simulink model "PubIfDecisionLM_MDL"  (R2020b)
settings: configuration reference "DspaceConfig" (kept outside this file)
PostLoadFcn:
  | if any(exist('dsrtsu_mdlpostloadfcn', 'file') ~= 0), dsrtsu_mdlpostloadfcn('Execute', bdroot); end
InitFcn:
  | , if any(exist('dsmpb_private', 'file') ~= 0), dsmpb_private('dsmpb_mdlclblib', 'Init', bdroot); end,
undefined symbols (not defined in the file or in its folder): OFM_OBJ_FUSIONTYPE_E, OFM_OBJ_MOVINGSTATE_E, OFM_OBJ_ORIENTATION_E, OFM_OBJ_TYPE_E, P_LM_Cyc, P_LM_EMLHistKapRcdBufSize, P_LM_EMLHistTrajBaseDis, P_LM_EMLHistTrajPNum, P_LM_EMLKapCorrMaxThre, P_LM_EMLMinKapThre, P_LM_EMLPathDisDiffThre, P_LM_EMLQuaFiltPar, P_LM_EMLTurnActKapThre, P_LM_EMLValidQuaThre, P_LM_FntPath1Disgap, P_LM_FntPath1MinDis, P_LM_FntPath1Timegap, P_LM_FntPath2Disgap, P_LM_FntPath2MinDis, P_LM_FntPath2Timegap, P_LM_FntPath3Disgap, P_LM_FntPath3MinDis, P_LM_FntPath3Timegap, P_LM_FusBLParFiltP, P_LM_FusEVDifC2Thre, P_LM_FusEVOPath1AllVSLDisThre, P_LM_FusEVOPath1AllVSLLostNumThre, P_LM_FusEVOPath1AllVSLQuaThre, P_LM_FusEVOPath1OTLFacNLC, P_LM_FusOTLQuaThre, P_LM_FusOTLSW, P_LM_FusParC0Index, P_LM_FusParC1Index, P_LM_FusParC2Index, P_LM_FusParC3Index, P_LM_FusVSLQuaThre, P_LM_FusVSLSW, P_LM_FusVSLValidSteerWheerAngThre, P_LM_FusVSLValidVxvThre, P_LM_LaneWidth, P_LM_OTLBufTPInfoEvaFactor, P_LM_OTLObjNum, P_LM_OTLObjSelectAgeThre, P_LM_OTLObjSelectDxAssessVx, P_LM_OTLObjSelectDxThre, P_LM_OTLObjSelectVxThre, P_LM_OTLObjSelectVyAssessDx, P_LM_OTLObjSelectVyThre, P_LM_OTLTrajPntBaseDis, P_LM_OTLTrajStdThre, P_LM_VSLAvailLineNum, P_LM_VSLBLSDiffThre, P_LM_VSLBLSDisRatio, P_LM_VSLFusBLParFiltP_C1, P_LM_VSLFusBLParFiltP_C2, P_LM_VSLFusBLParFiltP_C3, P_LM_VSLFusBLParFiltP_Quality, P_LM_VSLHistTrajBaseDis, P_LM_VSLHistTrajPNum, P_LM_VSLLCC0diff ... (+18)
libraries: simulink x145, LM_LIB x43
(part 17 of 24)

== system PubIfDecisionLM_MDL/Subsystem2/LM_Fusion1/LM_FusRatioCalc/LM_Fusion_EVO/LM_FusEVORatioCalc/LM_Fusion_FntPathK/LM_FusEVOFntPath1/LM_FUS_EVOFEMLKAdju ==
  LM_EMLFntPath1Quality : Inport
  DIR_LC2LeValid : Inport  Port=2
  DIR_LC2RigValid : Inport  Port=3
  vxvRefMs : Inport  Port=4
  LM_FusEVOFntPath1EMLKBefAdju : Inport  Port=5
  LM_FusEVOFntPath1VSLKBefAdju : Inport  Port=6
  LM_FusEVOFntPath1OTLKBefAdju : Inport  Port=7
  Add : Sum
  Compare To Zero : simulink/Logic and Bit Operations/Compare To Zero  relop===  OutDataTypeStr=boolean
  Constant : Constant  Value=0.000001  OutDataTypeStr=single
  Constant1 : Constant  OutDataTypeStr=single
  Constant2 : Constant  Value=10  OutDataTypeStr=single
  Constant3 : Constant  Value=6  OutDataTypeStr=single
  Constant4 : Constant  Value=0.6  OutDataTypeStr=single
  Constant5 : Constant  Value=0.45  OutDataTypeStr=single
  Constant7 : Constant  Value=0.6
  Divide : Product  Inputs=*/
  Divide1 : Product  Inputs=*/
  Logical Operator : Logic  AllPortsSameDT=off  OutDataTypeStr=boolean
  Logical Operator1 : Logic  AllPortsSameDT=off  OutDataTypeStr=boolean
  Logical Operator2 : Logic  Operator=OR  AllPortsSameDT=off  OutDataTypeStr=boolean
  Logical Operator3 : Logic  Operator=NOT  AllPortsSameDT=off  OutDataTypeStr=boolean
  Logical Operator4 : Logic  AllPortsSameDT=off  OutDataTypeStr=boolean
  Max : MinMax  Function=max  Inputs=2
  Max1 : MinMax  Function=max  Inputs=2
  Product : Product
  Product1 : Product
  Relational Operator1 : RelationalOperator  OutDataTypeStr=boolean  RndMeth=Simplest
  Relational Operator2 : RelationalOperator  OutDataTypeStr=boolean  RndMeth=Simplest
  Relational Operator3 : RelationalOperator  OutDataTypeStr=boolean  RndMeth=Simplest
  Subtract : Sum  Inputs=+-
  Switch{,1..4} (5 alike) : Switch  Criteria=u2 ~= 0
  LM_FusEVOFntPath1EMLK : Outport
  LM_FusEVOFntPath1VSLK : Outport  Port=2
  LM_FusEVOFntPath1OTLK : Outport  Port=3
  wires:
  Relational Operator2/1 -> Logical Operator1/2
  Relational Operator1/1 -> Logical Operator/2
  Logical Operator4/1 -> Logical Operator/1, Logical Operator1/1
  Constant7/1 -> Relational Operator3/2
  Max1/1 -> Switch2/1
  Constant5/1 -> Max1/2
  Switch2/1 -> Switch1/3
  Max/1 -> Switch1/1
  LM_FusEVOFntPath1EMLKBefAdju/1 -> Switch2/3, Max1/1, Max/1
  Constant4/1 -> Max/2
  Logical Operator1/1 -> Switch4/2, Switch3/2, Switch2/2
  Constant3/1 -> Relational Operator2/2
  Logical Operator/1 -> Switch1/2
  Constant2/1 -> Relational Operator1/2
  vxvRefMs/1 -> Relational Operator1/1, Relational Operator2/1
  LM_EMLFntPath1Quality/1 -> Relational Operator3/1
  Switch1/1 -> LM_FusEVOFntPath1EMLK/1, Subtract/2  "LM_FusEOFntPath1EMLK"
  DIR_LC2LeValid/1 -> Logical Operator2/1
  DIR_LC2RigValid/1 -> Logical Operator2/2
  Logical Operator2/1 -> Logical Operator3/1
  Logical Operator3/1 -> Logical Operator4/1
  Relational Operator3/1 -> Logical Operator4/2
  LM_FusEVOFntPath1VSLKBefAdju/1 -> Add/1, Switch3/3, Divide/1
  LM_FusEVOFntPath1OTLKBefAdju/1 -> Divide1/1, Switch4/3, Add/2
  Add/1 -> Switch/3, Compare To Zero/1
  Compare To Zero/1 -> Switch/2
  Constant/1 -> Switch/1
  Switch/1 -> Divide/2, Divide1/2
  Constant1/1 -> Subtract/1
  Subtract/1 -> Product1/1, Product/1
  Divide/1 -> Product/2
  Product/1 -> Switch3/1
  Product1/1 -> Switch4/1
  Divide1/1 -> Product1/2
  Switch3/1 -> LM_FusEVOFntPath1VSLK/1  "LM_FusEVOFntPath1VSLK"
  Switch4/1 -> LM_FusEVOFntPath1OTLK/1  "LM_FusEVOFntPath1OTLK"

== system PubIfDecisionLM_MDL/Subsystem2/LM_Fusion1/LM_FusRatioCalc/LM_Fusion_EVO/LM_FusEVORatioCalc/LM_Fusion_FntPathK/LM_FusEVOFntPath1/LM_FusEVOFntPath1AllEML ==
  Action Port : ActionPort  ActionPortLabel=elseif(u1 ==2)
  Constant : Constant  OutDataTypeStr=single
  Constant1 : Constant  Value=0  OutDataTypeStr=single
  Constant2 : Constant  Value=0  OutDataTypeStr=single
  LM_FusEVOFntPath1EMLK : Outport
  LM_FusEVOFntPath1VSLK : Outport  Port=2
  LM_FusEVOFntPath1OTLK : Outport  Port=3
  wires:
  Constant/1 -> LM_FusEVOFntPath1EMLK/1
  Constant2/1 -> LM_FusEVOFntPath1OTLK/1
  Constant1/1 -> LM_FusEVOFntPath1VSLK/1

== system PubIfDecisionLM_MDL/Subsystem2/LM_Fusion1/LM_FusRatioCalc/LM_Fusion_EVO/LM_FusEVORatioCalc/LM_Fusion_FntPathK/LM_FusEVOFntPath1/LM_FusEVOFntPath1AllVSL ==
  Action Port : ActionPort  ActionPortLabel=if(u1 == 1)
  Constant : Constant  Value=0  OutDataTypeStr=single
  Constant1 : Constant  OutDataTypeStr=single
  Constant2 : Constant  Value=0  OutDataTypeStr=single
  LM_FusEVOFntPath1EMLK : Outport
  LM_FusEVOFntPath1VSLK : Outport  Port=2
  LM_FusEVOFntPath1OTLK : Outport  Port=3
  wires:
  Constant/1 -> LM_FusEVOFntPath1EMLK/1
  Constant1/1 -> LM_FusEVOFntPath1VSLK/1
  Constant2/1 -> LM_FusEVOFntPath1OTLK/1

== system PubIfDecisionLM_MDL/Subsystem2/LM_Fusion1/LM_FusRatioCalc/LM_Fusion_EVO/LM_FusEVORatioCalc/LM_Fusion_FntPathK/LM_FusEVOFntPath1/LM_FusEVO_AllVSLJudge ==
  note: 0 Fus
      | 1 All VSL
      | 2 All EML
  note: 完全用车道线场景：当车道线很好的时候可以完全用车道线，否则为了增加道路模型鲁棒性对三个道路模型加权平均
      | 1. 丢失车道数<=1
      | 2. 车道线质量大于0.65
      | 3. 第一段道路模型距离-VSL基础距离<=8m
  LM_VSLBaseDis : Inport
  LM_ComLineLostNum : Inport  Port=2
  LM_FntPath1Dis : Inport  Port=3
  DIR_TurnLeftValid : Inport  Port=4
  DIR_TurnRightValid : Inport  Port=5
  LM_VSLFntPath1Quality : Inport  Port=6
  Constant : Constant  Value=P_LM_FusEVOPath1AllVSLLostNumThre  OutDataTypeStr=uint8
  Constant1 : Constant  Value=P_LM_FusEVOPath1AllVSLQuaThre  OutDataTypeStr=single
  Constant2 : Constant  Value=P_LM_FusEVOPath1AllVSLDisThre  OutDataTypeStr=single
  Constant3 : Constant  OutDataTypeStr=uint8
  Constant4 : Constant  Value=0  OutDataTypeStr=uint8
  Constant5 : Constant  Value=2  OutDataTypeStr=uint8
  Logical Operator : Logic  Inputs=3  AllPortsSameDT=off  OutDataTypeStr=boolean
  Logical Operator1 : Logic  Operator=OR  AllPortsSameDT=off  OutDataTypeStr=boolean
  Relational Operator : RelationalOperator  Operator=<=  OutDataTypeStr=boolean  RndMeth=Simplest
  Relational Operator1 : RelationalOperator  OutDataTypeStr=boolean  RndMeth=Simplest
  Relational Operator2 : RelationalOperator  Operator=<=  OutDataTypeStr=boolean  RndMeth=Simplest
  Subtract : Sum  Inputs=+-
  Switch : Switch  Criteria=u2 ~= 0
  Switch1 : Switch  Criteria=u2 ~= 0
  LM_FusEVOFusType : Outport
  wires:
  LM_ComLineLostNum/1 -> Relational Operator/1
  Constant/1 -> Relational Operator/2
  LM_VSLFntPath1Quality/1 -> Relational Operator1/1
  Constant1/1 -> Relational Operator1/2
  LM_VSLBaseDis/1 -> Subtract/2
  LM_FntPath1Dis/1 -> Subtract/1
  Subtract/1 -> Relational Operator2/1
  Constant2/1 -> Relational Operator2/2
  Relational Operator1/1 -> Logical Operator/1
  Relational Operator/1 -> Logical Operator/2
  Relational Operator2/1 -> Logical Operator/3
  Logical Operator/1 -> Switch1/2  "LM_FusEVOAllVSLflg"
  DIR_TurnLeftValid/1 -> Logical Operator1/1
  DIR_TurnRightValid/1 -> Logical Operator1/2
  Logical Operator1/1 -> Switch/2  "LM_FusEVOAllEMLflg"
  Switch/1 -> LM_FusEVOFusType/1  "LM_FusEVOFusType"
  Constant3/1 -> Switch1/1
  Constant4/1 -> Switch1/3
  Switch1/1 -> Switch/3
  Constant5/1 -> Switch/1

== system PubIfDecisionLM_MDL/Subsystem2/LM_Fusion1/LM_FusRatioCalc/LM_Fusion_EVO/LM_FusEVORatioCalc/LM_Fusion_FntPathK/LM_FusEVOFntPath2/If Action Subsystem ==
  Action Port : ActionPort  ActionPortLabel=if(u1 == 1)
  Constant : Constant  Value=0  OutDataTypeStr=single
  Constant1 : Constant  OutDataTypeStr=single
  Constant2 : Constant  Value=0  OutDataTypeStr=single
  LM_FusEVOFntPath2EMLK : Outport
  LM_FusEVOFntPath2VSLK : Outport  Port=2
  LM_FusEVOFntPath2OTLK : Outport  Port=3
  wires:
  Constant2/1 -> LM_FusEVOFntPath2OTLK/1
  Constant1/1 -> LM_FusEVOFntPath2VSLK/1
  Constant/1 -> LM_FusEVOFntPath2EMLK/1

== system PubIfDecisionLM_MDL/Subsystem2/LM_Fusion1/LM_FusRatioCalc/LM_Fusion_EVO/LM_FusEVORatioCalc/LM_Fusion_FntPathK/LM_FusEVOFntPath2/If Action Subsystem1 ==
  LM_EMLFntPath2Quality : Inport
  LM_VSLFntPath2Quality : Inport  Port=2
  LM_OTLFntPath2Qulity : Inport  Port=3
  vxvRefMs : Inport  Port=4
  DIR_LC2LeValid : Inport  Port=5
  DIR_LC2RigValid : Inport  Port=6
  Action Port : ActionPort  ActionPortLabel=else
  LM_FusEVO_EMLFactor : Subsystem
  LM_FusEVO_OTLFactor : Subsystem
  LM_FusEVO_VSLFactor : Subsystem
  Subsystem : Subsystem
  LM_FusEVOFntPath2EMLK : Outport
  LM_FusEVOFntPath2VSLK : Outport  Port=2
  LM_FusEVOFntPath2OTLK : Outport  Port=3
  wires:
  Subsystem/1(LM_FusEVOFntPath2EMLK) -> LM_FusEVOFntPath2EMLK/1  "LM_FusEVOFntPath2EMLK"
  Subsystem/2(LM_FusEVOFntPath2VSLK) -> LM_FusEVOFntPath2VSLK/1
  Subsystem/3(LM_FusEVOFntPath2OTLK) -> LM_FusEVOFntPath2OTLK/1
  vxvRefMs/1 -> LM_FusEVO_EMLFactor/1(vxvRefMs)
  DIR_LC2LeValid/1 -> LM_FusEVO_OTLFactor/1(DIR_LC2LeValid), LM_FusEVO_EMLFactor/2(DIR_LC2LeValid)
  DIR_LC2RigValid/1 -> LM_FusEVO_OTLFactor/2(DIR_LC2RigValid), LM_FusEVO_EMLFactor/3(DIR_LC2RigValid)
  LM_FusEVO_EMLFactor/1(LM_FusEVOFntPath2EMLFac) -> Subsystem/1(LM_FusEVOFntPath2EMLFac)
  LM_FusEVO_VSLFactor/1(LM_FusEVOFntPath2VSLFac) -> Subsystem/2(LM_FusEVOFntPath2VSLFac)
  LM_FusEVO_OTLFactor/1(LM_FusEVOFntPath2OTLFac) -> Subsystem/3(LM_FusEVOFntPath2OTLFac)
  LM_EMLFntPath2Quality/1 -> Subsystem/4(LM_EMLFntPath2Quality)
  LM_VSLFntPath2Quality/1 -> Subsystem/5(LM_VSLFntPath2Quality)
  LM_OTLFntPath2Qulity/1 -> Subsystem/6(LM_OTLFntPath2Qulity)

== system PubIfDecisionLM_MDL/Subsystem2/LM_Fusion1/LM_FusRatioCalc/LM_Fusion_EVO/LM_FusEVORatioCalc/LM_Fusion_FntPathK/LM_FusEVOFntPath2/If Action Subsystem2 ==
  Action Port : ActionPort  ActionPortLabel=elseif(u1 == 2)
  Constant : Constant  OutDataTypeStr=single
  Constant1 : Constant  Value=0  OutDataTypeStr=single
  Constant2 : Constant  Value=0  OutDataTypeStr=single
  LM_FusEVOFntPath2EMLK : Outport
  LM_FusEVOFntPath2VSLK : Outport  Port=2
  LM_FusEVOFntPath2OTLK : Outport  Port=3
  wires:
  Constant/1 -> LM_FusEVOFntPath2EMLK/1
  Constant1/1 -> LM_FusEVOFntPath2VSLK/1
  Constant2/1 -> LM_FusEVOFntPath2OTLK/1

== system PubIfDecisionLM_MDL/Subsystem2/LM_Fusion1/LM_FusRatioCalc/LM_Fusion_EVO/LM_FusEVORatioCalc/LM_Fusion_FntPathK/LM_FusEVOFntPath2/LM_FusEVO_AllVSLJudge ==
  note: 完全用车道线场景：当车道线很好的时候可以完全用车道线，否则为了增加道路模型鲁棒性对三个道路模型加权平均
      | 1. 丢失车道数<=1
      | 2. 车道线质量大于0.65
      | 3. 第一段道路模型距离-VSL基础距离<=8m
  note: 0 Fus
      | 1 All VSL
      | 2 All EML
  LM_ComLineLostNum : Inport
  DIR_TurnLeftValid : Inport  Port=2
  DIR_TurnRightValid : Inport  Port=3
  LM_VSLBaseDis : Inport  Port=4
  LM_FntPath2Dis : Inport  Port=5
  LM_VSLFntPath2Quality : Inport  Port=6
  Constant : Constant  OutDataTypeStr=uint8
  Constant1 : Constant  Value=0.5  OutDataTypeStr=single
  Constant2 : Constant  OutDataTypeStr=uint8
  Constant3 : Constant  Value=0  OutDataTypeStr=uint8
  Constant4 : Constant  Value=8  OutDataTypeStr=single
  Constant5 : Constant  Value=2  OutDataTypeStr=uint8
  Logical Operator : Logic  Inputs=3  AllPortsSameDT=off  OutDataTypeStr=boolean
  Logical Operator1 : Logic  Operator=OR  AllPortsSameDT=off  OutDataTypeStr=boolean
  Relational Operator : RelationalOperator  Operator=<=  OutDataTypeStr=boolean  RndMeth=Simplest
  Relational Operator1 : RelationalOperator  OutDataTypeStr=boolean  RndMeth=Simplest
  Relational Operator2 : RelationalOperator  Operator=<=  OutDataTypeStr=boolean  RndMeth=Simplest
  Subtract : Sum  Inputs=+-
  Switch : Switch  Criteria=u2 ~= 0
  Switch1 : Switch  Criteria=u2 ~= 0
  LM_FusEVOFntPath2FusType : Outport
  wires:
  Logical Operator/1 -> Switch1/2  "LM_FusEVOAllVSLflg"
  Relational Operator/1 -> Logical Operator/2
  Relational Operator1/1 -> Logical Operator/1
  Constant1/1 -> Relational Operator1/2
  LM_VSLFntPath2Quality/1 -> Relational Operator1/1
  Constant/1 -> Relational Operator/2
  LM_ComLineLostNum/1 -> Relational Operator/1
  Constant5/1 -> Switch/1
  Logical Operator1/1 -> Switch/2  "LM_FusEVOAllEMLflg"
  DIR_TurnRightValid/1 -> Logical Operator1/2
  DIR_TurnLeftValid/1 -> Logical Operator1/1
  Switch/1 -> LM_FusEVOFntPath2FusType/1  "LM_FusEVOFntPath2FusType"
  Switch1/1 -> Switch/3
  Constant2/1 -> Switch1/1
  Constant3/1 -> Switch1/3
  Subtract/1 -> Relational Operator2/1
  Constant4/1 -> Relational Operator2/2
  LM_FntPath2Dis/1 -> Subtract/1
  LM_VSLBaseDis/1 -> Subtract/2
  Relational Operator2/1 -> Logical Operator/3

== system PubIfDecisionLM_MDL/Subsystem2/LM_Fusion1/LM_FusRatioCalc/LM_Fusion_EVO/LM_FusEVORatioCalc/LM_Fusion_FntPathK/LM_FusEVOFntPath3/If Action Subsystem ==
  Action Port : ActionPort  ActionPortLabel=if(u1 == 1)
  Constant : Constant  Value=0  OutDataTypeStr=single
  Constant1 : Constant  OutDataTypeStr=single
  Constant2 : Constant  Value=0  OutDataTypeStr=single
  LM_FusEVOFntPath3EMLK : Outport
  LM_FusEVOFntPath3VSLK : Outport  Port=2
  LM_FusEVOFntPath3OTLK : Outport  Port=3
  wires:
  Constant2/1 -> LM_FusEVOFntPath3OTLK/1
  Constant1/1 -> LM_FusEVOFntPath3VSLK/1
  Constant/1 -> LM_FusEVOFntPath3EMLK/1

== system PubIfDecisionLM_MDL/Subsystem2/LM_Fusion1/LM_FusRatioCalc/LM_Fusion_EVO/LM_FusEVORatioCalc/LM_Fusion_FntPathK/LM_FusEVOFntPath3/If Action Subsystem1 ==
  LM_EMLFntPath3Quality : Inport
  LM_VSLFntPath3Quality : Inport  Port=2
  LM_OTLFntPath3Qulity : Inport  Port=3
  vxvRefMs : Inport  Port=4
  DIR_LC2LeValid : Inport  Port=5
  DIR_LC2RigValid : Inport  Port=6
  Action Port : ActionPort  ActionPortLabel=else
  LM_FusEVO_EMLFactor : Subsystem
  LM_FusEVO_OTLFactor : Subsystem
  LM_FusEVO_VSLFactor : Subsystem
  Subsystem : Subsystem
  LM_FusEVOFntPath3EMLK : Outport
  LM_FusEVOFntPath3VSLK : Outport  Port=2
  LM_FusEVOFntPath3OTLK : Outport  Port=3
  wires:
  DIR_LC2RigValid/1 -> LM_FusEVO_EMLFactor/3(DIR_LC2RigValid), LM_FusEVO_OTLFactor/2(DIR_LC2RigValid)
  DIR_LC2LeValid/1 -> LM_FusEVO_EMLFactor/2(DIR_LC2LeValid), LM_FusEVO_OTLFactor/1(DIR_LC2LeValid)
  vxvRefMs/1 -> LM_FusEVO_EMLFactor/1(vxvRefMs)
  LM_FusEVO_OTLFactor/1(LM_FusEVOFntPath3OTLFac) -> Subsystem/3(LM_FusEVOFntPath3OTLFac)
  LM_FusEVO_VSLFactor/1(LM_FusEVOFntPath3VSLFac) -> Subsystem/2(LM_FusEVOFntPath3VSLFac)
  LM_FusEVO_EMLFactor/1(LM_FusEVOFntPath3EMLFac) -> Subsystem/1(LM_FusEVOFntPath3EMLFac)
  Subsystem/2(LM_FusEVOFntPath3VSLK) -> LM_FusEVOFntPath3VSLK/1
  Subsystem/3(LM_FusEVOFntPath3OTLK) -> LM_FusEVOFntPath3OTLK/1
  Subsystem/1(LM_FusEVOFntPath3EMLK) -> LM_FusEVOFntPath3EMLK/1
  LM_EMLFntPath3Quality/1 -> Subsystem/4(LM_EMLFntPath3Quality)
  LM_VSLFntPath3Quality/1 -> Subsystem/5(LM_VSLFntPath3Quality)
  LM_OTLFntPath3Qulity/1 -> Subsystem/6(LM_OTLFntPath3Qulity)

== system PubIfDecisionLM_MDL/Subsystem2/LM_Fusion1/LM_FusRatioCalc/LM_Fusion_EVO/LM_FusEVORatioCalc/LM_Fusion_FntPathK/LM_FusEVOFntPath3/If Action Subsystem2 ==
  Action Port : ActionPort  ActionPortLabel=elseif(u1 == 2)
  Constant : Constant  OutDataTypeStr=single
  Constant1 : Constant  Value=0  OutDataTypeStr=single
  Constant2 : Constant  Value=0  OutDataTypeStr=single
  LM_FusEVOFntPath3EMLK : Outport
  LM_FusEVOFntPath3VSLK : Outport  Port=2
  LM_FusEVOFntPath3OTLK : Outport  Port=3
  wires:
  Constant/1 -> LM_FusEVOFntPath3EMLK/1
  Constant1/1 -> LM_FusEVOFntPath3VSLK/1
  Constant2/1 -> LM_FusEVOFntPath3OTLK/1

== system PubIfDecisionLM_MDL/Subsystem2/LM_Fusion1/LM_FusRatioCalc/LM_Fusion_EVO/LM_FusEVORatioCalc/LM_Fusion_FntPathK/LM_FusEVOFntPath3/LM_FusEVO_AllVSLJudge ==
  note: 完全用车道线场景：当车道线很好的时候可以完全用车道线，否则为了增加道路模型鲁棒性对三个道路模型加权平均
      | 1. 丢失车道数<=1
      | 2. 车道线质量大于0.65
      | 3. 第一段道路模型距离-VSL基础距离<=8m
  LM_ComLineLostNum : Inport
  DIR_TurnLeftValid : Inport  Port=2
  DIR_TurnRightValid : Inport  Port=3
  LM_VSLFntPath3Quality : Inport  Port=4
  Constant : Constant  OutDataTypeStr=uint8
  Constant1 : Constant  Value=0.45  OutDataTypeStr=single
  Constant2 : Constant  OutDataTypeStr=uint8
  Constant3 : Constant  Value=0  OutDataTypeStr=uint8
  Constant5 : Constant  Value=2  OutDataTypeStr=uint8
  Logical Operator : Logic  AllPortsSameDT=off  OutDataTypeStr=boolean
  Logical Operator1 : Logic  Operator=OR  AllPortsSameDT=off  OutDataTypeStr=boolean
  Relational Operator : RelationalOperator  Operator=<=  OutDataTypeStr=boolean  RndMeth=Simplest
  Relational Operator1 : RelationalOperator  OutDataTypeStr=boolean  RndMeth=Simplest
  Switch : Switch  Criteria=u2 ~= 0
  Switch1 : Switch  Criteria=u2 ~= 0
  LM_FusEVOFntPath3FusType : Outport
  wires:
  Logical Operator/1 -> Switch1/2  "LM_FusEVOAllVSLflg"
  Relational Operator/1 -> Logical Operator/2
  Relational Operator1/1 -> Logical Operator/1
  Constant1/1 -> Relational Operator1/2
  LM_VSLFntPath3Quality/1 -> Relational Operator1/1
  Constant/1 -> Relational Operator/2
  LM_ComLineLostNum/1 -> Relational Operator/1
  Switch1/1 -> Switch/3
  DIR_TurnRightValid/1 -> Logical Operator1/2
  Logical Operator1/1 -> Switch/2  "LM_FusEVOAllEMLflg"
  Constant5/1 -> Switch/1
  DIR_TurnLeftValid/1 -> Logical Operator1/1
  Constant2/1 -> Switch1/1
  Constant3/1 -> Switch1/3
  Switch/1 -> LM_FusEVOFntPath3FusType/1  "LM_FusEVOFntPath3FusType"

== system PubIfDecisionLM_MDL/Subsystem2/LM_Fusion1/LM_Fus_BLConnectivityCheck/LM_Fus_BLFntPahtConnectivityCheck/LM_Fus_BLFntPahtConnectivityCheck/LM_Fus_BLFntPath2Info/LM_Fus_BLFntPath2C0Adju/LM_Fus_BLFntPaht1EndPosCalc ==
  LM_FusBLFntPath1C0 : Inport
  LM_FusBLFntPath1C1 : Inport  Port=2
  LM_FusBLFntPath1C2 : Inport  Port=3
  LM_FusBLFntPath1C3 : Inport  Port=4
  LM_FntPath1Dis : Inport  Port=5
  Add : Sum
  Add1 : Sum
  Add2 : Sum
  Math Function : Math  Operator=square  SaturateOnIntegerOverflow=on
  Product{,1..3} (4 alike) : Product
  LM_FusBLFntPaht1EndPosdy : Outport
  wires:
  LM_FusBLFntPath1C0/1 -> Add/1
  LM_FntPath1Dis/1 -> Product3/2, Math Function/1, Product/2
  LM_FusBLFntPath1C1/1 -> Product/1
  LM_FusBLFntPath1C2/1 -> Product1/1
  Math Function/1 -> Product3/1, Product1/2
  LM_FusBLFntPath1C3/1 -> Product2/2
  Product3/1 -> Product2/1
  Product/1 -> Add/2
  Add/1 -> Add1/1
  Product1/1 -> Add1/2
  Add1/1 -> Add2/1
  Product2/1 -> Add2/2
  Add2/1 -> LM_FusBLFntPaht1EndPosdy/1  "LM_FusBLFntPaht1EndPosdy"

== system PubIfDecisionLM_MDL/Subsystem2/LM_Fusion1/LM_Fus_BLConnectivityCheck/LM_Fus_BLFntPahtConnectivityCheck/LM_Fus_BLFntPahtConnectivityCheck/LM_Fus_BLFntPath2Info/LM_Fus_BLFntPath2C0Adju/LM_Fus_BLFntPath2C0Adju ==
  LM_FusBLFntPaht1EndPosdy : Inport
  LM_FusBLFntPaht2StartPosdy : Inport  Port=2
  LM_FusBLFntPath2C0BefAduj : Inport  Port=3
  Add : Sum
  Subtract : Sum  Inputs=+-
  LM_FusBLFntPath2C0Aduj : Outport
  wires:
  LM_FusBLFntPaht1EndPosdy/1 -> Subtract/1
  LM_FusBLFntPaht2StartPosdy/1 -> Subtract/2
  Subtract/1 -> Add/1
  LM_FusBLFntPath2C0BefAduj/1 -> Add/2
  Add/1 -> LM_FusBLFntPath2C0Aduj/1  "LM_FusBLFntPath2C0Aduj"

== system PubIfDecisionLM_MDL/Subsystem2/LM_Fusion1/LM_Fus_BLConnectivityCheck/LM_Fus_BLFntPahtConnectivityCheck/LM_Fus_BLFntPahtConnectivityCheck/LM_Fus_BLFntPath2Info/LM_Fus_BLFntPath2C0Adju/LM_Fus_BLFntPath2StartPosCalc ==
  LM_FntPath1Dis : Inport
  LM_FusBLFntPath2C1 : Inport  Port=2
  LM_FusBLFntPath2C2 : Inport  Port=3
  LM_FusBLFntPath2C3 : Inport  Port=4
  LM_FusBLFntPath2C0BefAduj : Inport  Port=5
  Add : Sum
  Add1 : Sum
  Add2 : Sum
  Math Function : Math  Operator=square  SaturateOnIntegerOverflow=on
  Product{,1..3} (4 alike) : Product
  LM_FusBLFntPaht2StartPosdy : Outport
  wires:
  Product/1 -> Add/2
  LM_FusBLFntPath2C3/1 -> Product2/2
  LM_FusBLFntPath2C2/1 -> Product1/1
  Product3/1 -> Product2/1
  Product2/1 -> Add2/2
  Add1/1 -> Add2/1
  Add/1 -> Add1/1
  Product1/1 -> Add1/2
  Add2/1 -> LM_FusBLFntPaht2StartPosdy/1  "LM_FusBLFntPaht2StartPosdy"
  Math Function/1 -> Product3/1, Product1/2
  LM_FusBLFntPath2C1/1 -> Product/1
  LM_FusBLFntPath2C0BefAduj/1 -> Add/1
  LM_FntPath1Dis/1 -> Product3/2, Math Function/1, Product/2

== system PubIfDecisionLM_MDL/Subsystem2/LM_Fusion1/LM_Fus_BLConnectivityCheck/LM_Fus_BLFntPahtConnectivityCheck/LM_Fus_BLFntPahtConnectivityCheck/LM_Fus_BLFntPath3Info/LM_Fus_BLFntPath2C0Adju/LM_Fus_BLFntPaht2EndPosCalc ==
  LM_FusBLFntPath2C0 : Inport
  LM_FusBLFntPath2C1 : Inport  Port=2
  LM_FusBLFntPath2C2 : Inport  Port=3
  LM_FusBLFntPath2C3 : Inport  Port=4
  LM_FntPath2Dis : Inport  Port=5
  Add : Sum
  Add1 : Sum
  Add2 : Sum
  Math Function : Math  Operator=square  SaturateOnIntegerOverflow=on
  Product{,1..3} (4 alike) : Product
  LM_FusBLFntPaht2EndPosdy : Outport
  wires:
  LM_FusBLFntPath2C0/1 -> Add/1
  LM_FntPath2Dis/1 -> Product3/2, Math Function/1, Product/2
  LM_FusBLFntPath2C1/1 -> Product/1
  LM_FusBLFntPath2C2/1 -> Product1/1
  Math Function/1 -> Product3/1, Product1/2
  LM_FusBLFntPath2C3/1 -> Product2/2
  Product3/1 -> Product2/1
  Product/1 -> Add/2
  Add/1 -> Add1/1
  Product1/1 -> Add1/2
  Add1/1 -> Add2/1
  Product2/1 -> Add2/2
  Add2/1 -> LM_FusBLFntPaht2EndPosdy/1  "LM_FusBLFntPaht2EndPosdy"

== system PubIfDecisionLM_MDL/Subsystem2/LM_Fusion1/LM_Fus_BLConnectivityCheck/LM_Fus_BLFntPahtConnectivityCheck/LM_Fus_BLFntPahtConnectivityCheck/LM_Fus_BLFntPath3Info/LM_Fus_BLFntPath2C0Adju/LM_Fus_BLFntPath3C0Adju ==
  LM_FusBLFntPaht2EndPosdy : Inport
  LM_FusBLFntPaht3StartPosdy : Inport  Port=2
  LM_FusBLFntPath3C0BefAduj : Inport  Port=3
  Add : Sum
  Subtract : Sum  Inputs=+-
  LM_FusBLFntPath3C0Aduj : Outport
  wires:
  LM_FusBLFntPaht2EndPosdy/1 -> Subtract/1
  LM_FusBLFntPaht3StartPosdy/1 -> Subtract/2
  Subtract/1 -> Add/1
  LM_FusBLFntPath3C0BefAduj/1 -> Add/2
  Add/1 -> LM_FusBLFntPath3C0Aduj/1  "LM_FusBLFntPath3C0Aduj"

== system PubIfDecisionLM_MDL/Subsystem2/LM_Fusion1/LM_Fus_BLConnectivityCheck/LM_Fus_BLFntPahtConnectivityCheck/LM_Fus_BLFntPahtConnectivityCheck/LM_Fus_BLFntPath3Info/LM_Fus_BLFntPath2C0Adju/LM_Fus_BLFntPath3StartPosCalc ==
  LM_FntPath2Dis : Inport
  LM_FusBLFntPath3C1 : Inport  Port=2
  LM_FusBLFntPath3C2 : Inport  Port=3
  LM_FusBLFntPath3C3 : Inport  Port=4
  LM_FusBLFntPath3C0BefAduj : Inport  Port=5
  Add : Sum
  Add1 : Sum
  Add2 : Sum
  Math Function : Math  Operator=square  SaturateOnIntegerOverflow=on
  Product{,1..3} (4 alike) : Product
  LM_FusBLFntPaht3StartPosdy : Outport
  wires:
  Product/1 -> Add/2
  LM_FusBLFntPath3C3/1 -> Product2/2
  LM_FusBLFntPath3C2/1 -> Product1/1
  Product3/1 -> Product2/1
  Product2/1 -> Add2/2
  Add1/1 -> Add2/1
  Add/1 -> Add1/1
  Product1/1 -> Add1/2
  Add2/1 -> LM_FusBLFntPaht3StartPosdy/1  "LM_FusBLFntPaht3StartPosdy"
  Math Function/1 -> Product3/1, Product1/2
  LM_FusBLFntPath3C1/1 -> Product/1
  LM_FusBLFntPath3C0BefAduj/1 -> Add/1
  LM_FntPath2Dis/1 -> Product3/2, Math Function/1, Product/2

== system PubIfDecisionLM_MDL/Subsystem2/LM_Fusion1/LM_Fus_BLConnectivityCheck/LM_Fus_BLRearPahtConnectivityCheck/LM_Fus_BLRearPahtConnectivityCheck/LM_Fus_BLFntPath2Info/LM_Fus_BLFntPath2C0Adju/LM_Fus_BLFntPaht1EndPosCalc ==
  LM_FusBLFntPath1C0 : Inport
  LM_FusBLFntPath1C1 : Inport  Port=2
  LM_FusBLFntPath1C2 : Inport  Port=3
  LM_FusBLFntPath1C3 : Inport  Port=4
  LM_FntPath1Dis : Inport  Port=5
  Add : Sum
  Add1 : Sum
  Add2 : Sum
  Math Function : Math  Operator=square  SaturateOnIntegerOverflow=on
  Product{,1..3} (4 alike) : Product
  LM_FusBLFntPaht1EndPosdy : Outport
  wires:
  LM_FusBLFntPath1C0/1 -> Add/1
  LM_FntPath1Dis/1 -> Product3/2, Math Function/1, Product/2
  LM_FusBLFntPath1C1/1 -> Product/1
  LM_FusBLFntPath1C2/1 -> Product1/1
  Math Function/1 -> Product3/1, Product1/2
  LM_FusBLFntPath1C3/1 -> Product2/2
  Product3/1 -> Product2/1
  Product/1 -> Add/2
  Add/1 -> Add1/1
  Product1/1 -> Add1/2
  Add1/1 -> Add2/1
  Product2/1 -> Add2/2
  Add2/1 -> LM_FusBLFntPaht1EndPosdy/1  "LM_FusBLFntPaht1EndPosdy"

== system PubIfDecisionLM_MDL/Subsystem2/LM_Fusion1/LM_Fus_BLConnectivityCheck/LM_Fus_BLRearPahtConnectivityCheck/LM_Fus_BLRearPahtConnectivityCheck/LM_Fus_BLFntPath2Info/LM_Fus_BLFntPath2C0Adju/LM_Fus_BLFntPath2C0Adju ==
  LM_FusBLFntPaht1EndPosdy : Inport
  LM_FusBLFntPaht2StartPosdy : Inport  Port=2
  LM_FusBLFntPath2C0BefAduj : Inport  Port=3
  Add : Sum
  Subtract : Sum  Inputs=+-
  LM_FusBLFntPath2C0Aduj : Outport
  wires:
  LM_FusBLFntPaht1EndPosdy/1 -> Subtract/1
  LM_FusBLFntPaht2StartPosdy/1 -> Subtract/2
  Subtract/1 -> Add/1
  LM_FusBLFntPath2C0BefAduj/1 -> Add/2
  Add/1 -> LM_FusBLFntPath2C0Aduj/1  "LM_FusBLFntPath2C0Aduj"

== system PubIfDecisionLM_MDL/Subsystem2/LM_Fusion1/LM_Fus_BLConnectivityCheck/LM_Fus_BLRearPahtConnectivityCheck/LM_Fus_BLRearPahtConnectivityCheck/LM_Fus_BLFntPath2Info/LM_Fus_BLFntPath2C0Adju/LM_Fus_BLFntPath2StartPosCalc ==
  LM_FntPath1Dis : Inport
  LM_FusBLFntPath2C1 : Inport  Port=2
  LM_FusBLFntPath2C2 : Inport  Port=3
  LM_FusBLFntPath2C3 : Inport  Port=4
  LM_FusBLFntPath2C0BefAduj : Inport  Port=5
  Add : Sum
  Add1 : Sum
  Add2 : Sum
  Math Function : Math  Operator=square  SaturateOnIntegerOverflow=on
  Product{,1..3} (4 alike) : Product
  LM_FusBLFntPaht2StartPosdy : Outport
  wires:
  Product/1 -> Add/2
  LM_FusBLFntPath2C3/1 -> Product2/2
  LM_FusBLFntPath2C2/1 -> Product1/1
  Product3/1 -> Product2/1
  Product2/1 -> Add2/2
  Add1/1 -> Add2/1
  Add/1 -> Add1/1
  Product1/1 -> Add1/2
  Add2/1 -> LM_FusBLFntPaht2StartPosdy/1  "LM_FusBLFntPaht2StartPosdy"
  Math Function/1 -> Product3/1, Product1/2
  LM_FusBLFntPath2C1/1 -> Product/1
  LM_FusBLFntPath2C0BefAduj/1 -> Add/1
  LM_FntPath1Dis/1 -> Product3/2, Math Function/1, Product/2

== system PubIfDecisionLM_MDL/Subsystem2/LM_Fusion1/LM_Fus_BLConnectivityCheck/LM_Fus_BLRearPahtConnectivityCheck/LM_Fus_BLRearPahtConnectivityCheck/LM_Fus_BLFntPath3Info/LM_Fus_BLRearPath3C0Adju/LM_Fus_BLFntPaht2EndPosCalc ==
  LM_FusBLFntPath2C0 : Inport
  LM_FusBLFntPath2C1 : Inport  Port=2
  LM_FusBLFntPath2C2 : Inport  Port=3
  LM_FusBLFntPath2C3 : Inport  Port=4
  LM_FntPath2Dis : Inport  Port=5
  Add : Sum
  Add1 : Sum
  Add2 : Sum
  Math Function : Math  Operator=square  SaturateOnIntegerOverflow=on
  Product{,1..3} (4 alike) : Product
  LM_FusBLFntPaht2EndPosdy : Outport
  wires:
  LM_FusBLFntPath2C0/1 -> Add/1
  LM_FntPath2Dis/1 -> Product3/2, Math Function/1, Product/2
  LM_FusBLFntPath2C1/1 -> Product/1
  LM_FusBLFntPath2C2/1 -> Product1/1
  Math Function/1 -> Product3/1, Product1/2
  LM_FusBLFntPath2C3/1 -> Product2/2
  Product3/1 -> Product2/1
  Product/1 -> Add/2
  Add/1 -> Add1/1
  Product1/1 -> Add1/2
  Add1/1 -> Add2/1
  Product2/1 -> Add2/2
  Add2/1 -> LM_FusBLFntPaht2EndPosdy/1  "LM_FusBLFntPaht2EndPosdy"

== system PubIfDecisionLM_MDL/Subsystem2/LM_Fusion1/LM_Fus_BLConnectivityCheck/LM_Fus_BLRearPahtConnectivityCheck/LM_Fus_BLRearPahtConnectivityCheck/LM_Fus_BLFntPath3Info/LM_Fus_BLRearPath3C0Adju/LM_Fus_BLFntPath3C0Adju ==
  LM_FusBLFntPaht2EndPosdy : Inport
  LM_FusBLFntPaht3StartPosdy : Inport  Port=2
  LM_FusBLFntPath3C0BefAduj : Inport  Port=3
  Add : Sum
  Subtract : Sum  Inputs=+-
  LM_FusBLFntPath3C0Check : Outport
  wires:
  LM_FusBLFntPaht2EndPosdy/1 -> Subtract/1
  LM_FusBLFntPaht3StartPosdy/1 -> Subtract/2
  Subtract/1 -> Add/1
  LM_FusBLFntPath3C0BefAduj/1 -> Add/2
  Add/1 -> LM_FusBLFntPath3C0Check/1  "LM_FusBLFntPath3C0Check"

== system PubIfDecisionLM_MDL/Subsystem2/LM_Fusion1/LM_Fus_BLConnectivityCheck/LM_Fus_BLRearPahtConnectivityCheck/LM_Fus_BLRearPahtConnectivityCheck/LM_Fus_BLFntPath3Info/LM_Fus_BLRearPath3C0Adju/LM_Fus_BLFntPath3StartPosCalc ==
  LM_FntPath2Dis : Inport
  LM_FusBLFntPath3C1 : Inport  Port=2
  LM_FusBLFntPath3C2 : Inport  Port=3
  LM_FusBLFntPath3C3 : Inport  Port=4
  LM_FusBLFntPath3C0BefAduj : Inport  Port=5
  Add : Sum
  Add1 : Sum
  Add2 : Sum
  Math Function : Math  Operator=square  SaturateOnIntegerOverflow=on
  Product{,1..3} (4 alike) : Product
  LM_FusBLFntPaht3StartPosdy : Outport
  wires:
  Product/1 -> Add/2
  LM_FusBLFntPath3C3/1 -> Product2/2
  LM_FusBLFntPath3C2/1 -> Product1/1
  Product3/1 -> Product2/1
  Product2/1 -> Add2/2
  Add1/1 -> Add2/1
  Add/1 -> Add1/1
  Product1/1 -> Add1/2
  Add2/1 -> LM_FusBLFntPaht3StartPosdy/1  "LM_FusBLFntPaht3StartPosdy"
  Math Function/1 -> Product3/1, Product1/2
  LM_FusBLFntPath3C1/1 -> Product/1
  LM_FusBLFntPath3C0BefAduj/1 -> Add/1
  LM_FntPath2Dis/1 -> Product3/2, Math Function/1, Product/2

== system PubIfDecisionLM_MDL/Subsystem2/LM_OTL/LM_OTL_MovObjTrajRecord3/LM_OTL_BufTPCC/Subsystem/LM_OTLHostBufCoordinateConvert/If Action Subsystem/For Each Subsystem ==
  LM_OTLOffsetX : Inport
  LM_OTLOffsetY : Inport  Port=2
  LM_OTLOffsetAng : Inport  Port=3
  LM_OTLBufE1DxVectK1 : Inport  Port=4  Partition=on  PartitionDimension=1  PartitionWidth=1  PartitionOffset=0
  LM_OTLBufE1DyVectK1 : Inport  Port=5  Partition=on  PartitionDimension=1  PartitionWidth=1  PartitionOffset=0
  LM_OTLBufE2DxVectK1 : Inport  Port=6  Partition=on  PartitionDimension=1  PartitionWidth=1  PartitionOffset=0
  LM_OTLBufE2DyVectK1 : Inport  Port=7  Partition=on  PartitionDimension=1  PartitionWidth=1  PartitionOffset=0
  For Each : ForEach  DisableCoverage=on
  LM_VSL_BufE1Convert : Subsystem
  LM_VSL_BufE2Convert : Subsystem
  LM_OTLBufE1DxVectK1Adju : Outport  ConcatenationDimension=1
  LM_OTLBufE1DyVectK1Adju : Outport  Port=2  ConcatenationDimension=1
  LM_OTLBufE2DxVectK1Adju : Outport  Port=3  ConcatenationDimension=1
  LM_OTLBufE2DyVectK1Adju : Outport  Port=4  ConcatenationDimension=1
  wires:
  LM_OTLBufE2DxVectK1/1 -> LM_VSL_BufE2Convert/1(LM_OTLBufE2DxVectK1)
  LM_OTLBufE2DyVectK1/1 -> LM_VSL_BufE2Convert/2(LM_OTLBufE2DyVectK1)
  LM_OTLBufE1DxVectK1/1 -> LM_VSL_BufE1Convert/1(LM_OTLBufE1DxVectK1)
  LM_OTLBufE1DyVectK1/1 -> LM_VSL_BufE1Convert/2(LM_OTLBufE1DyVectK1)
  LM_VSL_BufE2Convert/1(LM_OTLBufE2DxVectK1Adju) -> LM_OTLBufE2DxVectK1Adju/1
  LM_VSL_BufE2Convert/2(LM_OTLBufE2DyVectK1Adju) -> LM_OTLBufE2DyVectK1Adju/1
  LM_VSL_BufE1Convert/2(LM_OTLBufE1DyVectK1Adju) -> LM_OTLBufE1DyVectK1Adju/1
  LM_VSL_BufE1Convert/1(LM_OTLBufE1DxVectK1Adju) -> LM_OTLBufE1DxVectK1Adju/1
  LM_OTLOffsetAng/1 -> LM_VSL_BufE1Convert/5(LM_EgoVehOffsetAng), LM_VSL_BufE2Convert/5(LM_EgoVehOffsetAng)
  LM_OTLOffsetY/1 -> LM_VSL_BufE1Convert/4(LM_EgoVehOffsetY), LM_VSL_BufE2Convert/4(LM_EgoVehOffsetY)
  LM_OTLOffsetX/1 -> LM_VSL_BufE1Convert/3(LM_EgoVehOffsetX), LM_VSL_BufE2Convert/3(LM_EgoVehOffsetX)

== system PubIfDecisionLM_MDL/Subsystem2/LM_OTL/LM_OTL_MovObjTrajRecord3/LM_OTL_BufTPCC/Subsystem/LM_OTLLeBufCoordinateConvert/If Action Subsystem/For Each Subsystem ==
  LM_OTLOffsetX : Inport
  LM_OTLOffsetY : Inport  Port=2
  LM_OTLOffsetAng : Inport  Port=3
  LM_OTLBufL1DxVectK1 : Inport  Port=4  Partition=on  PartitionDimension=1  PartitionWidth=1  PartitionOffset=0
  LM_OTLBufL1DyVectK1 : Inport  Port=5  Partition=on  PartitionDimension=1  PartitionWidth=1  PartitionOffset=0
  LM_OTLBufL2DxVectK1 : Inport  Port=6  Partition=on  PartitionDimension=1  PartitionWidth=1  PartitionOffset=0
  LM_OTLBufL2DyVectK1 : Inport  Port=7  Partition=on  PartitionDimension=1  PartitionWidth=1  PartitionOffset=0
  For Each : ForEach  DisableCoverage=on
  LM_OTL_BufL1Convert : Subsystem
  LM_VSL_BufL2Convert : Subsystem
  LM_OTLBufL1DxVectK1Adju : Outport  ConcatenationDimension=1
  LM_OTLBufL1DyVectK1Adju : Outport  Port=2  ConcatenationDimension=1
  LM_OTLBufL2DxVectK1Adju : Outport  Port=3  ConcatenationDimension=1
  LM_OTLBufL2DyVectK1Adju : Outport  Port=4  ConcatenationDimension=1
  wires:
  LM_OTLBufL2DxVectK1/1 -> LM_VSL_BufL2Convert/1(LM_OTLBufL2DxVectK1)
  LM_OTLBufL2DyVectK1/1 -> LM_VSL_BufL2Convert/2(LM_OTLBufL2DyVectK1)
  LM_OTLBufL1DxVectK1/1 -> LM_OTL_BufL1Convert/1(LM_OTLBufL1DxVectK1)
  LM_OTLBufL1DyVectK1/1 -> LM_OTL_BufL1Convert/2(LM_OTLBufL1DyVectK1)
  LM_VSL_BufL2Convert/1(LM_OTLBufL2DxVectK1Adju) -> LM_OTLBufL2DxVectK1Adju/1
  LM_VSL_BufL2Convert/2(LM_OTLBufL2DyVectK1Adju) -> LM_OTLBufL2DyVectK1Adju/1
  LM_OTL_BufL1Convert/2(LM_OTLBufL1DyVectK1Adju) -> LM_OTLBufL1DyVectK1Adju/1
  LM_OTL_BufL1Convert/1(LM_OTLBufL1DxVectK1Adju) -> LM_OTLBufL1DxVectK1Adju/1
  LM_OTLOffsetAng/1 -> LM_OTL_BufL1Convert/5(LM_EgoVehOffsetAng), LM_VSL_BufL2Convert/5(LM_EgoVehOffsetAng)
  LM_OTLOffsetY/1 -> LM_OTL_BufL1Convert/4(LM_EgoVehOffsetY), LM_VSL_BufL2Convert/4(LM_EgoVehOffsetY)
  LM_OTLOffsetX/1 -> LM_OTL_BufL1Convert/3(LM_EgoVehOffsetX), LM_VSL_BufL2Convert/3(LM_EgoVehOffsetX)

== system PubIfDecisionLM_MDL/Subsystem2/LM_OTL/LM_OTL_MovObjTrajRecord3/LM_OTL_BufTPCC/Subsystem/LM_OTLRiBufCoordinateConvert/If Action Subsystem/For Each Subsystem ==
  LM_OTLOffsetX : Inport
  LM_OTLOffsetY : Inport  Port=2
  LM_OTLOffsetAng : Inport  Port=3
  LM_OTLBufR1DxVectK1 : Inport  Port=4  Partition=on  PartitionDimension=1  PartitionWidth=1  PartitionOffset=0
  LM_OTLBufR1DyVectK1 : Inport  Port=5  Partition=on  PartitionDimension=1  PartitionWidth=1  PartitionOffset=0
  LM_OTLBufR2DxVectK1 : Inport  Port=6  Partition=on  PartitionDimension=1  PartitionWidth=1  PartitionOffset=0
  LM_OTLBufR2DyVectK1 : Inport  Port=7  Partition=on  PartitionDimension=1  PartitionWidth=1  PartitionOffset=0
  For Each : ForEach  DisableCoverage=on
  LM_VSL_BufR1Convert : Subsystem
  LM_VSL_BufR2Convert : Subsystem
  LM_OTLBufR1DxVectK1Adju : Outport  ConcatenationDimension=1
  LM_OTLBufR1DyVectK1Adju : Outport  Port=2  ConcatenationDimension=1
  LM_OTLBufR2DxVectK1Adju : Outport  Port=3  ConcatenationDimension=1
  LM_OTLBufR2DyVectK1Adju : Outport  Port=4  ConcatenationDimension=1
  wires:
  LM_OTLBufR2DxVectK1/1 -> LM_VSL_BufR2Convert/1(LM_OTLBufR2DxVectK1)
  LM_OTLBufR2DyVectK1/1 -> LM_VSL_BufR2Convert/2(LM_OTLBufR2DyVectK1)
  LM_OTLBufR1DxVectK1/1 -> LM_VSL_BufR1Convert/1(LM_OTLBufR1DxVectK1)
  LM_OTLBufR1DyVectK1/1 -> LM_VSL_BufR1Convert/2(LM_OTLBufR1DyVectK1)
  LM_VSL_BufR2Convert/1(LM_OTLBufR2DxVectK1Adju) -> LM_OTLBufR2DxVectK1Adju/1
  LM_VSL_BufR2Convert/2(LM_OTLBufR2DyVectK1Adju) -> LM_OTLBufR2DyVectK1Adju/1
  LM_VSL_BufR1Convert/2(LM_OTLBufR1DyVectK1Adju) -> LM_OTLBufR1DyVectK1Adju/1
  LM_VSL_BufR1Convert/1(LM_OTLBufR1DxVectK1Adju) -> LM_OTLBufR1DxVectK1Adju/1
  LM_OTLOffsetAng/1 -> LM_VSL_BufR1Convert/5(LM_EgoVehOffsetAng), LM_VSL_BufR2Convert/5(LM_EgoVehOffsetAng)
  LM_OTLOffsetY/1 -> LM_VSL_BufR1Convert/4(LM_EgoVehOffsetY), LM_VSL_BufR2Convert/4(LM_EgoVehOffsetY)
  LM_OTLOffsetX/1 -> LM_VSL_BufR1Convert/3(LM_EgoVehOffsetX), LM_VSL_BufR2Convert/3(LM_EgoVehOffsetX)

== system PubIfDecisionLM_MDL/Subsystem2/LM_OTL/LM_OTL_MovObjTrajRecord3/LM_OTL_MovObjSelc/LM_OTL_MovObjInterestedSelc/LM_OTL_ObjSelcIndexCalc/LM_OTL_ObjSelcCalc/LM_OTL_HostObjSelc ==
  C_LM_ObjNum : Inport
  HostObjSelcDxInfo : Inport  Port=2
  LM_OTL_HostObj1Selc : Subsystem
  LM_OTL_HostObj2Selc : Subsystem
  HostObj1Index : Outport
  HostObj2Index : Outport  Port=2
  wires:
  LM_OTL_HostObj2Selc/1(LM_OTLLeObj2Index) -> HostObj2Index/1
  LM_OTL_HostObj1Selc/4(HostObj2SelcDxPro) -> LM_OTL_HostObj2Selc/3(HostObj2SelcDxPro)
  LM_OTL_HostObj1Selc/3(HostObj2SelcIndexPro) -> LM_OTL_HostObj2Selc/2(HostObj2SelcIndexPro)
  LM_OTL_HostObj1Selc/2(HostObj2SelcTrig) -> LM_OTL_HostObj2Selc/1(HostObj2SelcTrig)
  LM_OTL_HostObj1Selc/1(LM_OTLHostObj1Index) -> HostObj1Index/1
  C_LM_ObjNum/1 -> LM_OTL_HostObj1Selc/1(C_LM_ObjNum), LM_OTL_HostObj2Selc/5(C_LM_ObjNum)
  HostObjSelcDxInfo/1 -> LM_OTL_HostObj1Selc/2(In4), LM_OTL_HostObj2Selc/4(LM_OTL_HostObjSelcDxInfo)

== system PubIfDecisionLM_MDL/Subsystem2/LM_OTL/LM_OTL_MovObjTrajRecord3/LM_OTL_MovObjSelc/LM_OTL_MovObjInterestedSelc/LM_OTL_ObjSelcIndexCalc/LM_OTL_ObjSelcCalc/LM_OTL_LeObjSelc ==
  C_LM_ObjNum : Inport
  LeObjSelcDxInfo : Inport  Port=2
  LM_OTL_LeObj1Selc : Subsystem
  LM_OTL_LeObj2Selc : Subsystem
  LeObj1Index : Outport
  LeObj2Index : Outport  Port=2
  wires:
  LM_OTL_LeObj2Selc/1(LM_OTLLeObj2Index) -> LeObj2Index/1
  LM_OTL_LeObj1Selc/4(LeObj2SelcDxPro) -> LM_OTL_LeObj2Selc/3(LeObj2SelcDxPro)
  LM_OTL_LeObj1Selc/3(LeObj2SelcIndexPro) -> LM_OTL_LeObj2Selc/2(LeObj2SelcIndexPro)
  LM_OTL_LeObj1Selc/2(LeObj2SelcTrig) -> LM_OTL_LeObj2Selc/1(LeObj2SelcTrig)
  LM_OTL_LeObj1Selc/1(LM_OTLLeObj1Index) -> LeObj1Index/1
  C_LM_ObjNum/1 -> LM_OTL_LeObj1Selc/1(C_LM_ObjNum), LM_OTL_LeObj2Selc/5(C_LM_ObjNum)
  LeObjSelcDxInfo/1 -> LM_OTL_LeObj1Selc/2(LeObjSelcDxInfo), LM_OTL_LeObj2Selc/4(LeObjSelcDxInfo)

== system PubIfDecisionLM_MDL/Subsystem2/LM_OTL/LM_OTL_MovObjTrajRecord3/LM_OTL_MovObjSelc/LM_OTL_MovObjInterestedSelc/LM_OTL_ObjSelcIndexCalc/LM_OTL_ObjSelcCalc/LM_OTL_RigObjSelc ==
  C_LM_ObjNum : Inport
  RigObjSelcDxInfo : Inport  Port=2
  LM_OTL_RigObj1Selc : Subsystem
  LM_OTL_RigObj2Selc : Subsystem
  RigObj1Index : Outport
  RigObj2Index : Outport  Port=2
  wires:
  LM_OTL_RigObj2Selc/1(LM_OTLLeObj2Index) -> RigObj2Index/1
  LM_OTL_RigObj1Selc/4(RigObj2SelcDxPro) -> LM_OTL_RigObj2Selc/3(RigObj2SelcDxPro)
  LM_OTL_RigObj1Selc/3(RigObj2SelcIndexPro) -> LM_OTL_RigObj2Selc/2(RigObj2SelcIndexPro)
  LM_OTL_RigObj1Selc/2(RigObj2SelcTrig) -> LM_OTL_RigObj2Selc/1(RigObj2SelcTrig)
  LM_OTL_RigObj1Selc/1(LM_OTLLeObj1Index) -> RigObj1Index/1
  C_LM_ObjNum/1 -> LM_OTL_RigObj1Selc/1(C_LM_ObjNum), LM_OTL_RigObj2Selc/5(C_LM_ObjNum)
  RigObjSelcDxInfo/1 -> LM_OTL_RigObj1Selc/2(In4), LM_OTL_RigObj2Selc/4(LM_OTL_RigObjSelcDxInfo)

== system PubIfDecisionLM_MDL/Subsystem2/LM_OTL/LM_OTL_MovObjTrajRecord3/LM_OTL_MovObjSelc/LM_OTL_MovObjInterestedSelc/LM_OTL_ObjSelcIndexCalc/LM_OTL_ObjSelcInfoOpt/HostObjSelcInfoOpt ==
  ObjSelcDxInfo : Inport
  ObjSelcDyInfo : Inport  Port=2
  Compare To Constant3 : simulink/Logic and Bit Operations/Compare To Constant  relop=<=  const=1.75  OutDataTypeStr=boolean
  Compare To Constant4 : simulink/Logic and Bit Operations/Compare To Constant  relop=>  const=-1.75  OutDataTypeStr=boolean
  Compare To Zero1 : simulink/Logic and Bit Operations/Compare To Zero  relop===  OutDataTypeStr=boolean
  Constant3 : Constant  Value=255  OutDataTypeStr=single
  Constant6 : Constant  Value=255  OutDataTypeStr=single
  Logical Operator1 : Logic  AllPortsSameDT=off  OutDataTypeStr=boolean
  Switch11 : Switch  Criteria=u2 > Threshold
  Switch9 : Switch  Criteria=u2 ~= 0
  HostObjSlecDxInfo : Outport
  wires:
  Switch11/1 -> HostObjSlecDxInfo/1
  ObjSelcDxInfo/1 -> Switch9/1
  Logical Operator1/1 -> Switch9/2
  ObjSelcDyInfo/1 -> Compare To Constant3/1, Compare To Constant4/1
  Constant6/1 -> Switch9/3
  Compare To Constant4/1 -> Logical Operator1/2
  Switch9/1 -> Compare To Zero1/1, Switch11/3
  Constant3/1 -> Switch11/1
  Compare To Zero1/1 -> Switch11/2
  Compare To Constant3/1 -> Logical Operator1/1

== system PubIfDecisionLM_MDL/Subsystem2/LM_OTL/LM_OTL_MovObjTrajRecord3/LM_OTL_MovObjSelc/LM_OTL_MovObjInterestedSelc/LM_OTL_ObjSelcIndexCalc/LM_OTL_ObjSelcInfoOpt/LeObjSelcInfoOpt ==
  ObjSelcDxInfo : Inport
  ObjSelcDyInfo : Inport  Port=2
  Compare To Constant1 : simulink/Logic and Bit Operations/Compare To Constant  relop=<=  const=6  OutDataTypeStr=boolean
  Compare To Constant2 : simulink/Logic and Bit Operations/Compare To Constant  relop=>  const=1.45  OutDataTypeStr=boolean
  Compare To Zero : simulink/Logic and Bit Operations/Compare To Zero  relop===  OutDataTypeStr=boolean
  Constant : Constant  Value=255  OutDataTypeStr=single
  Constant5 : Constant  Value=255  OutDataTypeStr=single
  Logical Operator : Logic  AllPortsSameDT=off  OutDataTypeStr=boolean
  Switch4 : Switch  Criteria=u2 > Threshold
  Switch8 : Switch  Criteria=u2 ~= 0
  LeObjSelcDxInfo : Outport
  wires:
  ObjSelcDxInfo/1 -> Switch8/1
  Compare To Zero/1 -> Switch4/2
  Compare To Constant2/1 -> Logical Operator/2
  Switch8/1 -> Compare To Zero/1, Switch4/3
  Logical Operator/1 -> Switch8/2
  Switch4/1 -> LeObjSelcDxInfo/1
  ObjSelcDyInfo/1 -> Compare To Constant1/1, Compare To Constant2/1
  Constant5/1 -> Switch8/3
  Compare To Constant1/1 -> Logical Operator/1
  Constant/1 -> Switch4/1

== system PubIfDecisionLM_MDL/Subsystem2/LM_OTL/LM_OTL_MovObjTrajRecord3/LM_OTL_MovObjSelc/LM_OTL_MovObjInterestedSelc/LM_OTL_ObjSelcIndexCalc/LM_OTL_ObjSelcInfoOpt/RigObjSelcInfoOpt ==
  ObjSelcDxInfo : Inport
  ObjSelcDyInfo : Inport  Port=2
  Compare To Constant5 : simulink/Logic and Bit Operations/Compare To Constant  relop=>  const=-6  OutDataTypeStr=boolean
  Compare To Constant6 : simulink/Logic and Bit Operations/Compare To Constant  relop=<=  const=-1.45  OutDataTypeStr=boolean
  Compare To Zero2 : simulink/Logic and Bit Operations/Compare To Zero  relop===  OutDataTypeStr=boolean
  Constant4 : Constant  Value=255  OutDataTypeStr=single
  Constant7 : Constant  Value=255  OutDataTypeStr=single
  Logical Operator2 : Logic  AllPortsSameDT=off  OutDataTypeStr=boolean
  Switch10 : Switch  Criteria=u2 ~= 0
  Switch13 : Switch  Criteria=u2 > Threshold
  RigObjSlecDxInfo : Outport
  wires:
  ObjSelcDxInfo/1 -> Switch10/1
  Logical Operator2/1 -> Switch10/2
  Compare To Constant5/1 -> Logical Operator2/2
  Switch10/1 -> Compare To Zero2/1, Switch13/3
  Constant7/1 -> Switch10/3
  Constant4/1 -> Switch13/1
  Switch13/1 -> RigObjSlecDxInfo/1
  Compare To Zero2/1 -> Switch13/2
  Compare To Constant6/1 -> Logical Operator2/1
  ObjSelcDyInfo/1 -> Compare To Constant5/1, Compare To Constant6/1

== system PubIfDecisionLM_MDL/Subsystem2/LM_OTL/LM_OTL_MovObjTrajRecord3/LM_OTL_MovObjSelc/LM_OTL_MovObjInterestedSelc/LM_OTL_ObjSelcIndexCheck/HostObj1Check/If Action Subsystem ==
  Action Port : ActionPort  ActionPortLabel=if(u1 == 0)
  Constant : Constant  Value=0  OutDataTypeStr=int32
  LM_OTLHostObj1Index : Outport
  wires:
  Constant/1 -> LM_OTLHostObj1Index/1

== system PubIfDecisionLM_MDL/Subsystem2/LM_OTL/LM_OTL_MovObjTrajRecord3/LM_OTL_MovObjSelc/LM_OTL_MovObjInterestedSelc/LM_OTL_ObjSelcIndexCheck/HostObj1Check/If Action Subsystem1 ==
  HostObj1CheckInfo : Inport
  LM_OTL_MovObjValid : Inport  Port=2
  Object_DX : Inport  Port=3
  Action Port : ActionPort  ActionPortLabel=else
  Compare To Constant1 : simulink/Logic and Bit Operations/Compare To Constant  relop=<=  const=1.45  OutDataTypeStr=boolean
  Compare To Constant2 : simulink/Logic and Bit Operations/Compare To Constant  relop=>  const=-1.45  OutDataTypeStr=boolean
  Constant : Constant  Value=0  OutDataTypeStr=int32
  Logical Operator : Logic  AllPortsSameDT=off  OutDataTypeStr=boolean
  Logical Operator1 : Logic  AllPortsSameDT=off  OutDataTypeStr=boolean
  Multiport Switch : MultiPortSwitch  Inputs=1
  Multiport Switch1 : MultiPortSwitch  Inputs=1
  Switch : Switch  Criteria=u2 > Threshold
  LM_OTLHostObj1Index : Outport
  wires:
  Logical Operator1/1 -> Logical Operator/2
  Logical Operator/1 -> Switch/2
  Multiport Switch1/1 -> Compare To Constant2/1, Compare To Constant1/1
  Compare To Constant1/1 -> Logical Operator1/1
  Compare To Constant2/1 -> Logical Operator1/2
  Object_DX/1 -> Multiport Switch1/2
  LM_OTL_MovObjValid/1 -> Multiport Switch/2
  HostObj1CheckInfo/1 -> Multiport Switch1/1, Multiport Switch/1, Switch/1
  Switch/1 -> LM_OTLHostObj1Index/1
  Constant/1 -> Switch/3
  Multiport Switch/1 -> Logical Operator/1

== system PubIfDecisionLM_MDL/Subsystem2/LM_OTL/LM_OTL_MovObjTrajRecord3/LM_OTL_MovObjSelc/LM_OTL_MovObjInterestedSelc/LM_OTL_ObjSelcIndexCheck/HostObj2Check/If Action Subsystem ==
  Action Port : ActionPort  ActionPortLabel=if(u1 == 0)
  Constant : Constant  Value=0  OutDataTypeStr=int32
  LM_OTLHostObj2Index : Outport
  wires:
  Constant/1 -> LM_OTLHostObj2Index/1

== system PubIfDecisionLM_MDL/Subsystem2/LM_OTL/LM_OTL_MovObjTrajRecord3/LM_OTL_MovObjSelc/LM_OTL_MovObjInterestedSelc/LM_OTL_ObjSelcIndexCheck/HostObj2Check/If Action Subsystem1 ==
  LeObj1CheckInfo : Inport
  LM_OTL_MovObjValid : Inport  Port=2
  Object_DX : Inport  Port=3
  Action Port : ActionPort  ActionPortLabel=else
  Compare To Constant1 : simulink/Logic and Bit Operations/Compare To Constant  relop=<=  const=2  OutDataTypeStr=boolean
  Compare To Constant2 : simulink/Logic and Bit Operations/Compare To Constant  relop=>  const=-2  OutDataTypeStr=boolean
  Constant : Constant  Value=0  OutDataTypeStr=int32
  Logical Operator : Logic  AllPortsSameDT=off  OutDataTypeStr=boolean
  Logical Operator1 : Logic  AllPortsSameDT=off  OutDataTypeStr=boolean
  Multiport Switch : MultiPortSwitch  Inputs=1
  Multiport Switch1 : MultiPortSwitch  Inputs=1
  Switch : Switch  Criteria=u2 > Threshold
  LM_OTLLeObj1Index : Outport
  wires:
  Logical Operator1/1 -> Logical Operator/2
  Logical Operator/1 -> Switch/2
  Multiport Switch1/1 -> Compare To Constant2/1, Compare To Constant1/1
  Compare To Constant1/1 -> Logical Operator1/1
  Compare To Constant2/1 -> Logical Operator1/2
  Object_DX/1 -> Multiport Switch1/2
  LM_OTL_MovObjValid/1 -> Multiport Switch/2
  LeObj1CheckInfo/1 -> Multiport Switch1/1, Multiport Switch/1, Switch/1
  Switch/1 -> LM_OTLLeObj1Index/1
  Constant/1 -> Switch/3
  Multiport Switch/1 -> Logical Operator/1

== system PubIfDecisionLM_MDL/Subsystem2/LM_OTL/LM_OTL_MovObjTrajRecord3/LM_OTL_MovObjSelc/LM_OTL_MovObjInterestedSelc/LM_OTL_ObjSelcIndexCheck/LeObj1Check/If Action Subsystem ==
  Action Port : ActionPort  ActionPortLabel=if(u1 == 0)
  Constant : Constant  Value=0  OutDataTypeStr=int32
  LM_OTLLeObj1Index : Outport
  wires:
  Constant/1 -> LM_OTLLeObj1Index/1

== system PubIfDecisionLM_MDL/Subsystem2/LM_OTL/LM_OTL_MovObjTrajRecord3/LM_OTL_MovObjSelc/LM_OTL_MovObjInterestedSelc/LM_OTL_ObjSelcIndexCheck/LeObj1Check/If Action Subsystem1 ==
  LeObj1CheckInfo : Inport
  LM_OTL_MovObjValid : Inport  Port=2
  Object_DX : Inport  Port=3
  Action Port : ActionPort  ActionPortLabel=else
  Compare To Constant1 : simulink/Logic and Bit Operations/Compare To Constant  relop=<=  const=6  OutDataTypeStr=boolean
  Compare To Constant2 : simulink/Logic and Bit Operations/Compare To Constant  relop=>  const=1.45  OutDataTypeStr=boolean
  Constant : Constant  Value=0  OutDataTypeStr=int32
  Logical Operator : Logic  AllPortsSameDT=off  OutDataTypeStr=boolean
  Logical Operator1 : Logic  AllPortsSameDT=off  OutDataTypeStr=boolean
  Multiport Switch : MultiPortSwitch  Inputs=1
  Multiport Switch1 : MultiPortSwitch  Inputs=1
  Switch : Switch  Criteria=u2 > Threshold
  LM_OTLLeObj1Index : Outport
  wires:
  Logical Operator1/1 -> Logical Operator/2
  Logical Operator/1 -> Switch/2
  Multiport Switch1/1 -> Compare To Constant2/1, Compare To Constant1/1
  Compare To Constant1/1 -> Logical Operator1/1
  Compare To Constant2/1 -> Logical Operator1/2
  Object_DX/1 -> Multiport Switch1/2
  LM_OTL_MovObjValid/1 -> Multiport Switch/2
  LeObj1CheckInfo/1 -> Multiport Switch1/1, Multiport Switch/1, Switch/1
  Switch/1 -> LM_OTLLeObj1Index/1
  Constant/1 -> Switch/3
  Multiport Switch/1 -> Logical Operator/1

== system PubIfDecisionLM_MDL/Subsystem2/LM_OTL/LM_OTL_MovObjTrajRecord3/LM_OTL_MovObjSelc/LM_OTL_MovObjInterestedSelc/LM_OTL_ObjSelcIndexCheck/LeObj2Check/If Action Subsystem ==
  Action Port : ActionPort  ActionPortLabel=if(u1 == 0)
  Constant : Constant  Value=0  OutDataTypeStr=int32
  LM_OTLLeObj2Index : Outport
  wires:
  Constant/1 -> LM_OTLLeObj2Index/1

== system PubIfDecisionLM_MDL/Subsystem2/LM_OTL/LM_OTL_MovObjTrajRecord3/LM_OTL_MovObjSelc/LM_OTL_MovObjInterestedSelc/LM_OTL_ObjSelcIndexCheck/LeObj2Check/If Action Subsystem1 ==
  LeObj1CheckInfo : Inport
  LM_OTL_MovObjValid : Inport  Port=2
  Object_DX : Inport  Port=3
  Action Port : ActionPort  ActionPortLabel=else
  Compare To Constant1 : simulink/Logic and Bit Operations/Compare To Constant  relop=<=  const=6  OutDataTypeStr=boolean
  Compare To Constant2 : simulink/Logic and Bit Operations/Compare To Constant  relop=>  const=2  OutDataTypeStr=boolean
  Constant : Constant  Value=0  OutDataTypeStr=int32
  Logical Operator : Logic  AllPortsSameDT=off  OutDataTypeStr=boolean
  Logical Operator1 : Logic  AllPortsSameDT=off  OutDataTypeStr=boolean
  Multiport Switch : MultiPortSwitch  Inputs=1
  Multiport Switch1 : MultiPortSwitch  Inputs=1
  Switch : Switch  Criteria=u2 > Threshold
  LM_OTLLeObj2Index : Outport
  wires:
  Logical Operator1/1 -> Logical Operator/2
  Logical Operator/1 -> Switch/2
  Multiport Switch1/1 -> Compare To Constant2/1, Compare To Constant1/1
  Compare To Constant1/1 -> Logical Operator1/1
  Compare To Constant2/1 -> Logical Operator1/2
  Object_DX/1 -> Multiport Switch1/2
  LM_OTL_MovObjValid/1 -> Multiport Switch/2
  LeObj1CheckInfo/1 -> Multiport Switch1/1, Multiport Switch/1, Switch/1
  Switch/1 -> LM_OTLLeObj2Index/1
  Constant/1 -> Switch/3
  Multiport Switch/1 -> Logical Operator/1

== system PubIfDecisionLM_MDL/Subsystem2/LM_OTL/LM_OTL_MovObjTrajRecord3/LM_OTL_MovObjSelc/LM_OTL_MovObjInterestedSelc/LM_OTL_ObjSelcIndexCheck/RigObj1Check/If Action Subsystem ==
  Action Port : ActionPort  ActionPortLabel=if(u1 == 0)
  Constant : Constant  Value=0  OutDataTypeStr=int32
  LM_OTLLeObj1Index : Outport
  wires:
  Constant/1 -> LM_OTLLeObj1Index/1
